simulink model "Clock_Pendulum"  (R2023b)
settings: Solver=VariableStepAuto  StartTime=0.0  StopTime=10  MaxStep=0.01  RelTol=1e-3
model workspace (MAT data in the model file):
  L = 0.9939
  g = 9.81
  m = 1
settings Model: Creator=91839  LastModifiedBy=siva kumar
settings SolverCC: AlgebraicLoopSolver=TrustRegion
settings DataIOCC: ExternalInput=data  SaveFormat=Array  DSMLogging=off  ReturnWorkspaceOutputs=off
settings DebuggingCC: ReadBeforeWriteMsg=DisableAll  WriteAfterWriteMsg=DisableAll  WriteAfterReadMsg=DisableAll  MultiTaskDSMMsg=none  UnconnectedInputMsg=warning  UnconnectedOutputMsg=warning  UnconnectedLineMsg=warning
settings ModelReferenceCC: UpdateModelReferenceTargets=IfOutOfDate  EnableRefExpFcnMdlSchedulingChecks=on
settings SFSimCC: SFSimEcho=off  CustomCodeUndefinedFunction=UseInterfaceOnly

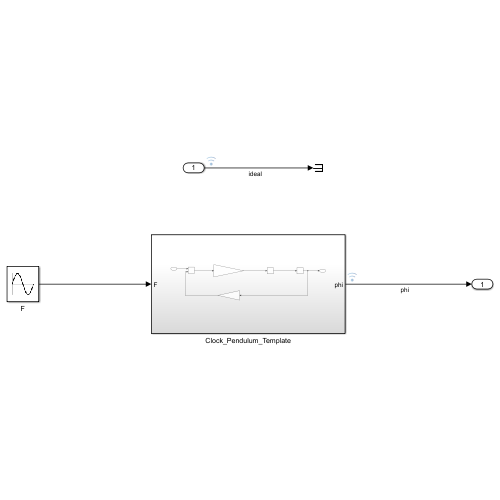
[thumbnail: Simulink's stored preview of the top-level diagram]
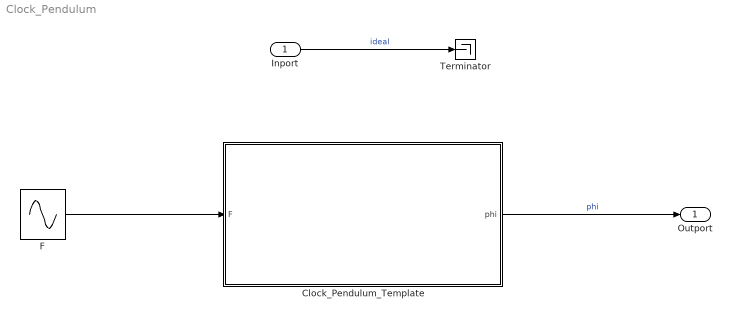
== system Clock_Pendulum ==
  Inport : Inport
  Clock_Pendulum_Template : Subsystem
  F : Sin  SampleTime=0
  Terminator : Terminator
  Outport : Outport
  wires:
  F/1 -> Clock_Pendulum_Template/1(F)
  Clock_Pendulum_Template/1(phi) -> Outport/1  "phi"
  Inport/1 -> Terminator/1  "ideal"

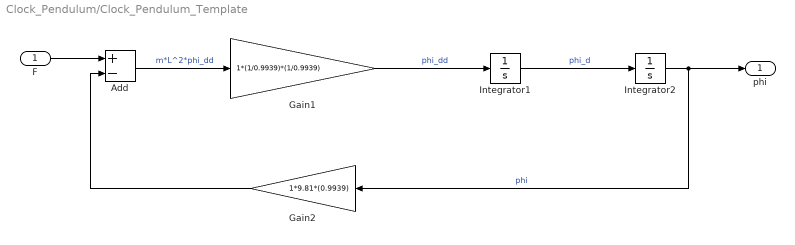
== system Clock_Pendulum/Clock_Pendulum_Template ==
  F : Inport
  Add : Sum  Inputs=+-
  Gain1 : Gain  Gain=1*(1/0.9939)*(1/0.9939)
  Gain2 : Gain  Gain=1*9.81*(0.9939)
  Integrator1 : Integrator
  Integrator2 : Integrator
  phi : Outport
  wires:
  Add/1 -> Gain1/1  "m*L^2*phi_dd"
  Gain1/1 -> Integrator1/1  "phi_dd"
  Integrator1/1 -> Integrator2/1  "phi_d"
  Integrator2/1 -> Gain2/1, phi/1  "phi"
  F/1 -> Add/1
  Gain2/1 -> Add/2
